simulink model "PlanarArmCL_LPV_Aug"  (R2025b)
settings: Solver=VariableStepAuto  StartTime=0.0  StopTime=10.0  RelTol=1e-3
undefined symbols (not defined in the file): JacobuInv, Kp, Kv, uss
libraries: RCTblocks x4, cstblocks x1
settings Model: Creator=d.alazard  LastModifiedBy=andre
settings SolverCC: AlgebraicLoopSolver=TrustRegion
settings DebuggingCC: AlgebraicLoopMsg=none  UnconnectedInputMsg=warning  UnconnectedOutputMsg=warning  UnconnectedLineMsg=warning
settings ModelReferenceCC: EnableRefExpFcnMdlSchedulingChecks=on
settings RTWCC: GPUComputeCapability=3.5  DLArmComputeVersion=19.05

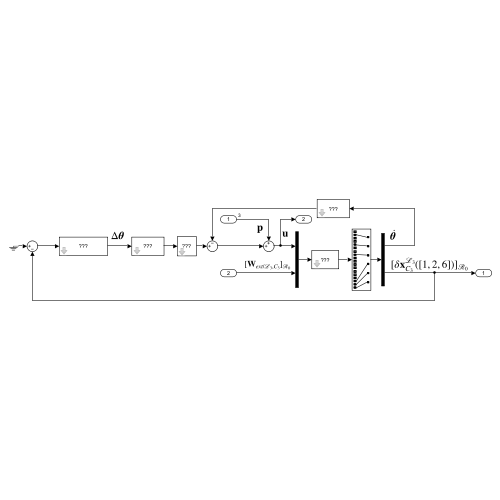
[thumbnail: Simulink's stored preview of the top-level diagram]
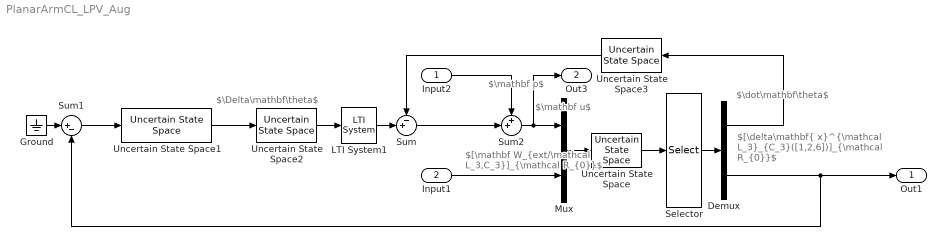
== system PlanarArmCL_LPV_Aug ==
  note: $\dot\mathbf\theta$
  note: $\mathbf u$
  note: $\Delta\mathbf\theta$
  note: $[\mathbf W_{ext/\mathcal L_3,C_3}]_{\mathcal R_{0}}$
  note: $\mathbf p$
  note: $[\delta\mathbf{ x}^{\mathcal L_3}_{C_3}([1,2,6])]_{\mathcal R_{0}}$
  Input2 : Inport  OutDataTypeStr=uint64  PortDimensions=3
  Input1 : Inport  Port=2
  Demux : Demux  Outputs=[3 3]
  Ground : Ground
  LTI System1 : cstblocks/LTI System  sys=F  IC=[]  PadeOrder=0
  Mux : Mux  Inputs=[3 3]
  Selector : Selector  InputPortWidth=18  IndexOptions=Index vector (dialog)  Indices=[2 5 8 16 17 18]  OutputSizes=1
  Sum : Sum  Inputs=-+|
  Sum1 : Sum  Inputs=|+-
  Sum2 : Sum  Inputs=++|
  Uncertain State Space : RCTblocks/Uncertain State Space  Tag=USS  USystem=Gfu  UValue=[]  X0=[]  uX0=[]
  Uncertain State Space1 : RCTblocks/Uncertain State Space  Tag=USS  USystem=uss(JacobuInv)  UValue=[]  X0=[]  uX0=[]
  Uncertain State Space2 : RCTblocks/Uncertain State Space  Tag=USS  USystem=uss(Kp)  UValue=[]  X0=[]  uX0=[]
  Uncertain State Space3 : RCTblocks/Uncertain State Space  Tag=USS  USystem=uss(Kv)  UValue=[]  X0=[]  uX0=[]
  Out1 : Outport
  Out3 : Outport  Port=2
  wires:
  Demux/1 -> Uncertain State Space3/1
  Uncertain State Space3/1 -> Sum/1
  Ground/1 -> Sum1/1
  Demux/2 -> Out1/1, Sum1/2
  Uncertain State Space1/1 -> Uncertain State Space2/1
  Sum1/1 -> Uncertain State Space1/1
  Mux/1 -> Uncertain State Space/1
  Input1/1 -> Mux/2
  Sum/1 -> Sum2/2
  Sum2/1 -> Out3/1, Mux/1
  Input2/1 -> Sum2/1
  Uncertain State Space2/1 -> LTI System1/1
  LTI System1/1 -> Sum/2
  Uncertain State Space/1 -> Selector/1
  Selector/1 -> Demux/1
